simulink model "LoadFlowA"  (R2016a)
settings: Solver=VariableStepAuto  SolverMode=SingleTasking  StartTime=0.0  StopTime=0.001  RelTol=1e-3
libraries: spsLoadFlowBusLib x3, spsThreePhaseParallelRLCLoadLib x3, spsThreePhasePISectionLineLib x3, spsSimplifiedSynchronousMachinepuUnitsLib x2, spspowerguiLib x1
settings Model: Creator=Asus  LastModifiedBy=User
settings DataIOCC: ReturnWorkspaceOutputs=on
settings DebuggingCC: SFUnexpectedBacktrackingDiag=error  SFNoUnconditionalDefaultTransitionDiag=error
settings SFSimCC: SimUseLocalCustomCode=on
settings RTWCC: RTWUseLocalCustomCode=on
settings GRTTargetCC: TargetLangStandard=C99 (ISO)
settings ConfigComp: CovMetricSettings=dwe  CovSaveCumulativeToWorkspaceVar=off  CovSaveSingleToWorkspaceVar=off  CovExternalEMLEnable=on

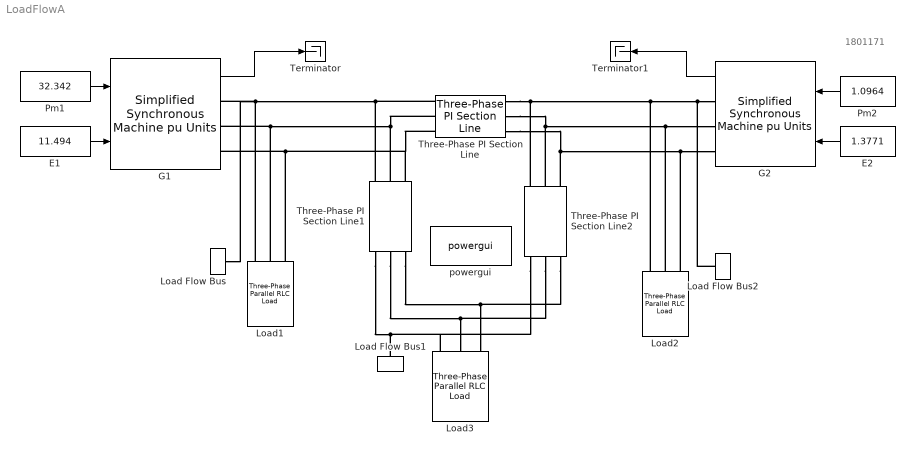
== system LoadFlowA ==
  note: 1801171
  E1 : Constant  Value=11.494
  E2 : Constant  Value=1.3771
  G1 : spsSimplifiedSynchronousMachinepuUnitsLib/Simplified Synchronous Machine pu Units  ConnectionType=3-wire Y  MechanicalLoad=Mechanical power Pm  MeasurementBus=off  NominalParameters=[100e6 150000 50]  Mechanical=[3.7 0 20]  InternalRL="[0.02  0.3]"  InitialConditions=[0 54.6549 38.0286 38.0286 38.0286 -31.1018 -151.102 88.8982]  IterativeDiscreteModel=Trapezoidal non iterative  TsBlock=-1  TsPowergui=0  LoadFlowParameters=[1,0,0,0,0]  Units=0  BusType=swing  Pref=0  Qref=0  Qmin=-Inf  Qmax=Inf  PLF=0  QLF=0
  G2 : spsSimplifiedSynchronousMachinepuUnitsLib/Simplified Synchronous Machine pu Units  ConnectionType=3-wire Y  MechanicalLoad=Mechanical power Pm  MeasurementBus=off  NominalParameters=[187e6 13800 60]  Mechanical=[3.7 0 20]  InternalRL="[0.02  0.3]"  InitialConditions=[0 10.7219 1.15917 1.15917 1.15917 -35.8978 -155.898 84.1022]  IterativeDiscreteModel=Trapezoidal non iterative  TsBlock=-1  TsPowergui=0  LoadFlowParameters=[1,0,0,0,0]  Units=0  BusType=PV  Pref=200000000  Qref=0  Qmin=-Inf  Qmax=Inf  PLF=0  QLF=0
  Load Flow Bus : spsLoadFlowBusLib/Load Flow Bus  LConnTagsString=a  Phases=single  Connectors=on one side  ID=BUS_1  Vbase=15e3  Vref=1.05  Vangle=0  VLF=1.05  VLFb=1  VLFc=1  angleLF=0  angleLFb=0  angleLFc=0
  Load Flow Bus1 : spsLoadFlowBusLib/Load Flow Bus  LConnTagsString=a  Phases=single  Connectors=on one side  ID=BUS_3  Vbase=15e3  Vref=0  Vangle=0  VLF=0.9767  VLFb=1  VLFc=1  angleLF=-3.643  angleLFb=0  angleLFc=0
  Load Flow Bus2 : spsLoadFlowBusLib/Load Flow Bus  LConnTagsString=a  Phases=single  Connectors=on one side  ID=BUS_2  Vbase=15e3  Vref=1.04  Vangle=0  VLF=1.04  VLFb=1  VLFc=1  angleLF=-0.6037  angleLFb=0  angleLFc=0
  Load1 : spsThreePhaseParallelRLCLoadLib/Three-Phase Parallel RLC Load  LConnTagsString=A|B|C  Configuration=Y (grounded)  NominalVoltage=(15000)*1.05  Vabc=[1e3 1e3 1e3]  Vabcp=[1e3 1e3 1e3]  NominalFrequency=50  UnbalancedPower=off  ActivePower=80000000  InductivePower=30000000  CapacitivePower=0  Pabc=[10e3 9e3 11e3]  QLabc=[100 90 110]  QCabc=[100 90 110]  Pabcp=[10e3 9e3 11e3]  QLabcp=[100 90 110]  QCabcp=[100 90 110]  Measurements=None  LoadType=constant PQ
  Load2 : spsThreePhaseParallelRLCLoadLib/Three-Phase Parallel RLC Load  LConnTagsString=A|B|C  Configuration=Y (grounded)  NominalVoltage=(15000)*1.04  Vabc=[1e3 1e3 1e3]  Vabcp=[1e3 1e3 1e3]  NominalFrequency=50  UnbalancedPower=off  ActivePower=50000000  InductivePower=25000000  CapacitivePower=0  Pabc=[10e3 9e3 11e3]  QLabc=[100 90 110]  QCabc=[100 90 110]  Pabcp=[10e3 9e3 11e3]  QLabcp=[100 90 110]  QCabcp=[100 90 110]  Measurements=None  LoadType=constant PQ
  Load3 : spsThreePhaseParallelRLCLoadLib/Three-Phase Parallel RLC Load  LConnTagsString=A|B|C  Configuration=Y (grounded)  NominalVoltage=(15000)*0.976655  Vabc=[1e3 1e3 1e3]  Vabcp=[1e3 1e3 1e3]  NominalFrequency=50  UnbalancedPower=off  ActivePower=400000000  InductivePower=250000000  CapacitivePower=0  Pabc=[10e3 9e3 11e3]  QLabc=[100 90 110]  QCabc=[100 90 110]  Pabcp=[10e3 9e3 11e3]  QLabcp=[100 90 110]  QCabcp=[100 90 110]  Measurements=None  LoadType=constant PQ
  Pm1 : Constant  Value=32.342
  Pm2 : Constant  Value=1.0964
  Terminator : Terminator
  Terminator1 : Terminator
  Three-Phase PI Section Line : spsThreePhasePISectionLineLib/Three-Phase PI Section Line  LConnTagsString=a|b|c  RConnTagsString=A|B|C  Length=1  Frequency=50  Resistances=[ 0.01*2.25 0.3864]  Inductances=[ (0.03*2.25)/(100*pi) 4.1264e-3]  Capacitances=[12.74e-9 7.751e-9]
  Three-Phase PI Section Line1 : spsThreePhasePISectionLineLib/Three-Phase PI Section Line  LConnTagsString=a|b|c  RConnTagsString=A|B|C  Length=1  Frequency=50  Resistances=[ 0.01*2.25 0.3864]  Inductances=[ (0.03*2.25)/(100*pi) 4.1264e-3]  Capacitances=[12.74e-9 7.751e-9]
  Three-Phase PI Section Line2 : spsThreePhasePISectionLineLib/Three-Phase PI Section Line  LConnTagsString=a|b|c  RConnTagsString=A|B|C  Length=1  Frequency=50  Resistances=[ 0.01*2.25 0.3864]  Inductances=[ (0.03*2.25)/(100*pi) 4.1264e-3]  Capacitances=[12.74e-9 7.751e-9]
  powergui : spspowerguiLib/powergui  Priority=1  SimulationMode=Continuous  SampleTime=50e-6  frequency=60  Iterations=50  frequencyindice=60  Pbase=100e6  ErrMax=1e-4  UnitsV=kV  UnitsW=MW  buscounter=0  FunctionMessages=off  echomessages=off  EnableUseOfTLC=off  CurrentSourceSwitches=off  DisableSnubberDevices=off  DisableRonSwitches=off  DisableVfSwitches=off  DisplayEquations=off  AutomaticDiscreteSolvers=off  SolverType=Tustin/Backward Euler (TBE)  Interpol=off  ExternalGateDelay=off  methode=off  Ts=100  x0status=blocks  SPID=on  SwTol=0  HookPort=off  NonlinearTolerance=1e-4  nMaxIteration=100  ContinueOnMaxIteration=off  RestoreLinks=warning  ResistiveCurrentMeasurement=off  Frange=[0:2:500]  Ylog=off  Xlog=on  ShowGrid=off  save=off  variable=ZData  structure=0  ZoomFFT=off  StartTime=0.0  cycles=1  DisplayStyle=1  fundamental=60  FreqAxis=off  MaxFrequency=1000  frequencyindicesteady=1  RmsSteady=1  display=off
  wires:
  E1/1 -> G1/2
  Pm1/1 -> G1/1
  G1/1 -> Terminator/1
  E2/1 -> G2/2
  Pm2/1 -> G2/1
  G2/1 -> Terminator1/1
  connections:
  Load1/LConn1 -- Load Flow Bus/LConn1 -- G1/RConn1 -- Three-Phase PI Section Line1/LConn1 -- Three-Phase PI Section Line/LConn1
  Load1/LConn2 -- Three-Phase PI Section Line1/LConn2 -- Three-Phase PI Section Line/LConn2 -- G1/RConn2
  Load1/LConn3 -- Three-Phase PI Section Line1/LConn3 -- Three-Phase PI Section Line/LConn3 -- G1/RConn3
  Three-Phase PI Section Line/RConn2 -- Three-Phase PI Section Line2/LConn2 -- Load2/LConn2 -- G2/RConn2
  Three-Phase PI Section Line/RConn1 -- Three-Phase PI Section Line2/LConn1 -- Load2/LConn1 -- G2/RConn1 -- Load Flow Bus2/LConn1
  Three-Phase PI Section Line/RConn3 -- Three-Phase PI Section Line2/LConn3 -- Load2/LConn3 -- G2/RConn3
  Three-Phase PI Section Line1/RConn1 -- Load3/LConn1 -- Three-Phase PI Section Line2/RConn1 -- Load Flow Bus1/LConn1
  Three-Phase PI Section Line1/RConn2 -- Load3/LConn2 -- Three-Phase PI Section Line2/RConn2
  Three-Phase PI Section Line1/RConn3 -- Load3/LConn3 -- Three-Phase PI Section Line2/RConn3
